simulink model "zero_to_hero_sect1to5"  (R2023a)
settings: Solver=FixedStepAuto  StartTime=0.0  StopTime=runtime  FixedStep=0.01  RelTol=1e-3
values from neighbouring files (symbols this model uses):
  b = 50    [zero_to_hero_sect10_script.m]    (also in zero_to_hero_sect1to5_script.m = 0.1; zero_to_hero_sect7to8_script.m = 10)
  F = 1.5    [zero_to_hero_sect1to5_script.m]
  k = 0.3    [zero_to_hero_sect1to5_script.m]    (also in zero_to_hero_sect7to8_script.m = 20)
  m = 1000    [zero_to_hero_sect10_script.m]    (also in zero_to_hero_sect1to5_script.m = 1; zero_to_hero_sect7to8_script.m = 1)
libraries: simulink x1
settings Model: Creator=fycce  LastModifiedBy=fycce

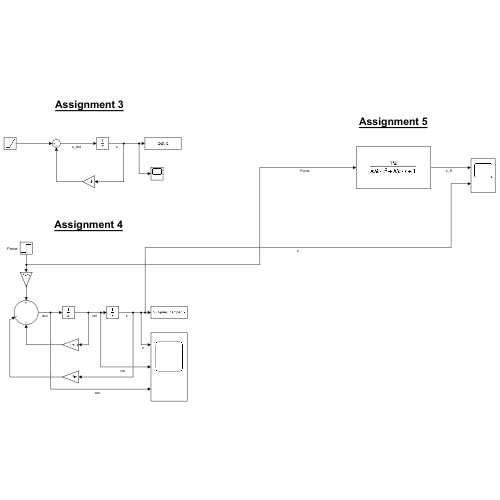
[thumbnail: Simulink's stored preview of the top-level diagram]
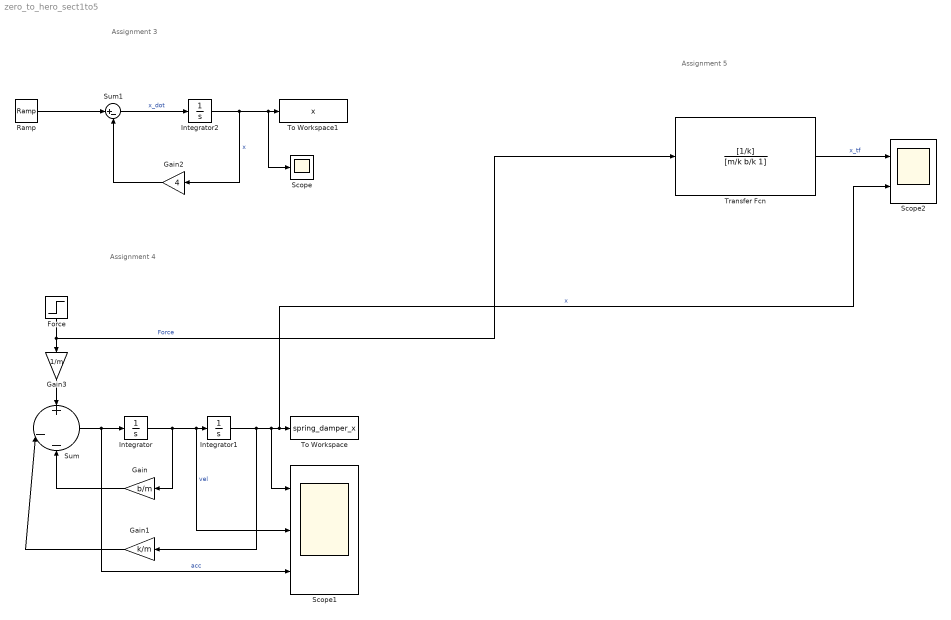
== system zero_to_hero_sect1to5 ==
  note: Assignment 4
  note: Assignment 3
  note: Assignment 5
  Force : Step  After=F  SampleTime=0
  Gain : Gain  Gain=b/m
  Gain1 : Gain  Gain=k/m
  Gain2 : Gain  Gain=4
  Gain3 : Gain  Gain=1/m
  Integrator : Integrator
  Integrator1 : Integrator
  Integrator2 : Integrator
  Ramp : simulink/Sources/Ramp  slope=1  start=0  InitialOutput=0
  Scope : Scope
  Scope1 : Scope  NumInputPorts=3
  Scope2 : Scope  NumInputPorts=2
  Sum : Sum  Inputs=+||||-||-
  Sum1 : Sum  Inputs=|+-
  To Workspace : ToWorkspace  VariableName=spring_damper_x  SaveFormat=Timeseries  SampleTime=-1
  To Workspace1 : ToWorkspace  VariableName=x  SaveFormat=Timeseries  SampleTime=-1
  Transfer Fcn : TransferFcn  Numerator=[1/k]  Denominator=[m/k b/k 1]
  wires:
  Sum/1 -> Integrator/1, Scope1/3  "acc"
  Integrator/1 -> Gain/1, Scope1/2, Integrator1/1  "vel"
  Integrator1/1 -> Gain1/1, Scope1/1, Scope2/2, To Workspace/1  "x"
  Gain/1 -> Sum/3
  Gain1/1 -> Sum/2
  Integrator2/1 -> Gain2/1, Scope/1, To Workspace1/1  "x"
  Gain2/1 -> Sum1/2
  Sum1/1 -> Integrator2/1  "x_dot"
  Ramp/1 -> Sum1/1
  Transfer Fcn/1 -> Scope2/1  "x_tf"
  Force/1 -> Gain3/1, Transfer Fcn/1  "Force"
  Gain3/1 -> Sum/1
